simulink model "q_heli3d_w_ads"  (Simulink 7.7)
settings: Solver=ode1  StartTime=0.0  StopTime=inf  FixedStep=0.002  RelTol=1e-3
values from neighbouring files (symbols this model uses):
  CAL_TIME = 1.0    (= 1)    [setup_ads_configuration.m]
  CAL_VEL = 0.02    [setup_ads_configuration.m]
  CMD_ELEV_POS_LIMIT_LOWER = elev_0*180/pi    (= -27.5)    [setup_lab_heli_3d.m]    (also in setup_lab_heli_3d_simple.m; setup_lab_heli_3d_various_controler.m; setup_lab_heli_3d_various_controler_with_Kalman_Filter.m)
  CMD_ELEV_POS_LIMIT_UPPER = -CMD_ELEV_POS_LIMIT_LOWER    (= 27.5)    [setup_lab_heli_3d.m]    (also in setup_lab_heli_3d_simple.m; setup_lab_heli_3d_various_controler.m; setup_lab_heli_3d_various_controler_with_Kalman_Filter.m)
  CMD_RATE_LIMIT = 45.0 * pi / 180    (= 0.785398163397)    [setup_lab_heli_3d.m]    (also in setup_lab_heli_3d_simple.m; setup_lab_heli_3d_various_controler.m; setup_lab_heli_3d_various_controler_with_Kalman_Filter.m)
  elev_0 = -27.5*pi/180    (= -0.479965544298)    [setup_lab_heli_3d.m]    (also in setup_lab_heli_3d_simple.m; setup_lab_heli_3d_various_controler.m; setup_lab_heli_3d_various_controler_with_Kalman_Filter.m)
  g = 9.81    [linnlsys.m]
  K = lqr(A,B,Q_x,Q_u)    [lab_init.m]    (also in setup_lab_heli_3d.m = zeros(2,6); setup_lab_heli_3d_various_controler.m = lqr( Ai, Bi, Q, R ); setup_lab_heli_3d_various_controler_with_Kalman_Filter.m = lqr( Ai, Bi, Q, R ))
  K_AMP = 3    [setup_lab_heli_3d.m]    (also in setup_lab_heli_3d_simple.m; setup_lab_heli_3d_various_controler.m; setup_lab_heli_3d_various_controler_with_Kalman_Filter.m)
  K_AMP_X = 3    [setup_lab_heli_3d.m]    (also in setup_lab_heli_3d_simple.m; setup_lab_heli_3d_various_controler.m; setup_lab_heli_3d_various_controler_with_Kalman_Filter.m)
  K_JOYSTICK_X = 40.0    (= 40)    [setup_lab_heli_3d.m]    (also in setup_lab_heli_3d_simple.m; setup_lab_heli_3d_various_controler.m; setup_lab_heli_3d_various_controler_with_Kalman_Filter.m)
  K_JOYSTICK_Y = 45.0    (= 45)    [setup_lab_heli_3d.m]    (also in setup_lab_heli_3d_simple.m; setup_lab_heli_3d_various_controler.m; setup_lab_heli_3d_various_controler_with_Kalman_Filter.m)
  kp = 225    [setup_ads_configuration.m]
  La = 26.0 * 0.0254    (= 0.6604)    [linnlsys.m]
  POS_HOME = 11 * 0.0254 / 2    (= 0.1397)    [setup_ads_configuration.m]
  SAT_INT_ERR_ELEV = 7.5    [setup_lab_heli_3d.m]    (also in setup_lab_heli_3d_simple.m; setup_lab_heli_3d_various_controler.m; setup_lab_heli_3d_various_controler_with_Kalman_Filter.m)
  SAT_INT_ERR_TRAVEL = 7.5    [setup_lab_heli_3d.m]    (also in setup_lab_heli_3d_simple.m; setup_lab_heli_3d_various_controler.m; setup_lab_heli_3d_various_controler_with_Kalman_Filter.m)
  V_MAX = 0.08    [setup_ads_configuration.m]
  VMAX_AMP = 24    [setup_lab_heli_3d.m]    (also in setup_lab_heli_3d_simple.m; setup_lab_heli_3d_various_controler.m; setup_lab_heli_3d_various_controler_with_Kalman_Filter.m)
  VMAX_AMP_X = 15    [setup_lab_heli_3d.m]    (also in setup_lab_heli_3d_simple.m; setup_lab_heli_3d_various_controler.m; setup_lab_heli_3d_various_controler_with_Kalman_Filter.m)
  VMAX_DAC = 10    [setup_lab_heli_3d.m]    (also in setup_lab_heli_3d_simple.m; setup_lab_heli_3d_various_controler.m; setup_lab_heli_3d_various_controler_with_Kalman_Filter.m)
  wcf = 2 * pi * 2.5    (= 15.7079632679)    [setup_ads_configuration.m]    (also in setup_lab_heli_3d.m = 125.663706144; setup_lab_heli_3d_simple.m = 125.663706144; setup_lab_heli_3d_various_controler.m = 125.663706144; setup_lab_heli_3d_various_controler_with_Kalman_Filter.m = 125.663706144)
  X_MAX = 11 * 0.024    (= 0.264)    [setup_ads_configuration.m]
  zetaf = 0.9    [setup_lab_heli_3d.m]    (also in setup_lab_heli_3d_simple.m; setup_lab_heli_3d_various_controler.m; setup_lab_heli_3d_various_controler_with_Kalman_Filter.m)
undefined symbols (not defined in the file or in its folder): CMD_TRAVEL_POS_LIMIT_LOWER, CMD_TRAVEL_POS_LIMIT_UPPER, HIL, K_EC_E, K_EC_P, K_EC_T, K_EC_X, Kf, Lw, m_b, m_f, m_w, qc_get_step_size, wcf_x
libraries: quarc_library x6, simulink_extras x5, simulink x4
settings Model: Creator=MLevis  LastModifiedBy=MLevis  SimulationMode=external  ExtModeTrigDuration=5000
settings SolverCC: PositivePriorityOrder=on
settings OptimizationCC: InitFltsAndDblsToZero=on
settings DebuggingCC: SaveWithParameterizedLinksMsg=none  StrictBusMsg=Warning
settings RTWCC: SystemTargetFile=quarc_windows.tlc  TemplateMakefile=quarc_default_tmf  Description=QUARC Win32 Target  ProcessScript=quarc_windows_make_rtw_hook
settings STFCustomTargetCC: TargetFcnLib=ansi_tfl_tmw.mat  TargetPreCompLibLocation=C:\PROGRA~3\QUARC\lib\2011a\windows\release  FunctionExecutionProfile=off  GeneratePreprocessorConditionals=Disable all  SystemTargetFile=quarc_windows.tlc
settings GRTTargetCC: TargetFcnLib=ansi_tfl_tmw.mat  TargetPreCompLibLocation=C:\PROGRA~3\QUARC\lib\2011a\windows\release  ParMdlRefBuildCompliant=off  CompOptLevelCompliant=off  MatFileLogging=off  ExtMode=on  ExtModeMexFile=quarc_comm

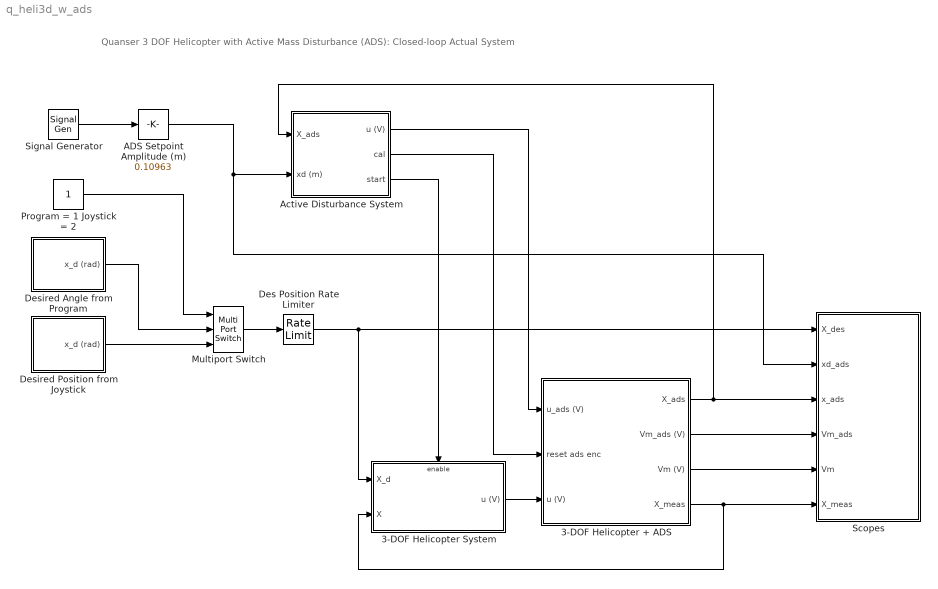
== system q_heli3d_w_ads ==
  note: Quanser 3 DOF Helicopter with Active Mass Disturbance (ADS):
      | Closed-loop Actual System
  3-DOF Helicopter + ADS : Subsystem
  3-DOF Helicopter System : Subsystem
  ADS Setpoint Amplitude (m) : simulink/Math Operations/Slider Gain  SystemSampleTime=-1  low=0  gain=0.10963  high=0.13
  Active Disturbance System : Subsystem
  Des Position Rate Limiter : RateLimiter  RisingSlewLimit=CMD_RATE_LIMIT  FallingSlewLimit=-CMD_RATE_LIMIT  SampleTimeMode=inherited
  Desired Angle from Program : Subsystem
  Desired Position from Joystick : Subsystem
  Multiport Switch : MultiPortSwitch  Inputs=2  zeroidx=off
  Program = 1 Joystick = 2 : Constant
  Scopes : Subsystem
  Signal Generator : SignalGenerator  WaveForm=square  Frequency=0.05
  wires:
  Signal Generator/1 -> ADS Setpoint Amplitude (m)/1
  ADS Setpoint Amplitude (m)/1 -> Scopes/2(xd_ads), Active Disturbance System/2(xd (m))
  Program = 1 Joystick = 2/1 -> Multiport Switch/1
  Desired Angle from Program/1(x_d (rad)) -> Multiport Switch/2
  Multiport Switch/1 -> Des Position Rate Limiter/1
  Desired Position from Joystick/1(x_d (rad)) -> Multiport Switch/3
  Des Position Rate Limiter/1 -> Scopes/1(X_des), 3-DOF Helicopter System/1(X_d)
  3-DOF Helicopter System/1(u (V)) -> 3-DOF Helicopter + ADS/3(u (V))
  Active Disturbance System/1(u (V)) -> 3-DOF Helicopter + ADS/1(u_ads (V))
  Active Disturbance System/2(cal) -> 3-DOF Helicopter + ADS/2(reset ads enc)
  3-DOF Helicopter + ADS/3(Vm (V)) -> Scopes/5(Vm)
  3-DOF Helicopter + ADS/4(X_meas) -> 3-DOF Helicopter System/2(X), Scopes/6(X_meas)
  3-DOF Helicopter + ADS/1(X_ads) -> Scopes/3(x_ads), Active Disturbance System/1(X_ads)
  Active Disturbance System/3(start) -> 3-DOF Helicopter System/Enable
  3-DOF Helicopter + ADS/2(Vm_ads (V)) -> Scopes/4(Vm_ads)

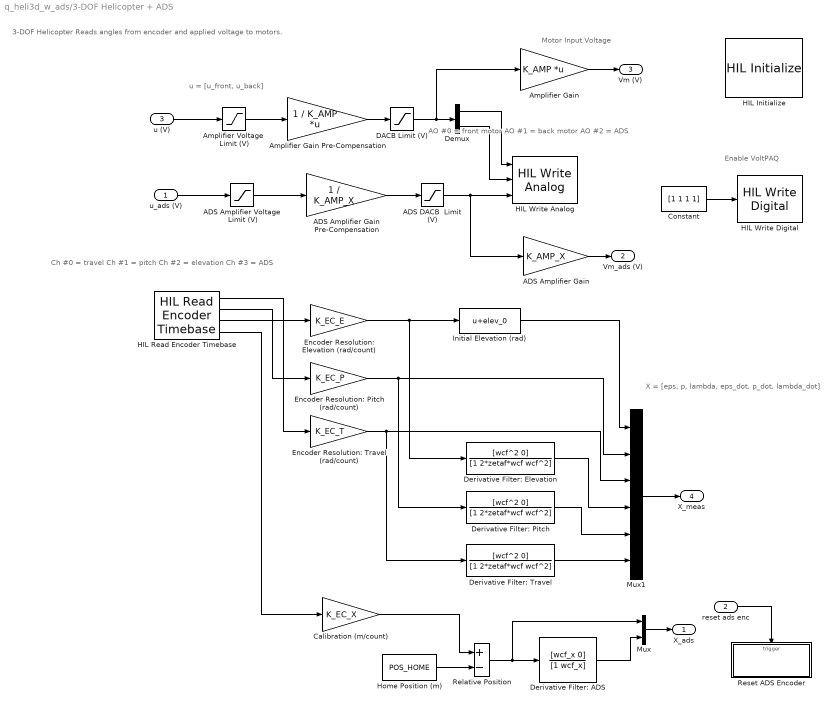
== system q_heli3d_w_ads/3-DOF Helicopter + ADS ==
  note: Enable VoltPAQ
  note: X = [eps, p, lambda, eps_dot, p_dot, lambda_dot]
  note: Ch #0 = travel
      | Ch #1 = pitch
      | Ch #2 = elevation
      | Ch #3 = ADS
  note: 3-DOF Helicopter
      | Reads angles from encoder and applied voltage to motors.
  note: Motor Input Voltage
  note: u = [u_front, u_back]
  note: AO #0 = front motor
      | AO #1 = back motor
      | AO #2 = ADS
  u_ads (V) : Inport
  reset ads enc : Inport  Port=2
  u (V) : Inport  Port=3
  ADS Amplifier Gain : Gain  Gain=K_AMP_X  SaturateOnIntegerOverflow=on  OutDataTypeStr=Inherit: Same as input  ParamDataTypeStr=Inherit: Same as input
  ADS Amplifier Gain Pre-Compensation : Gain  Gain=1 / K_AMP_X  SaturateOnIntegerOverflow=on  OutDataTypeStr=Inherit: Same as input  ParamDataTypeStr=Inherit: Same as input
  ADS Amplifier Voltage  Limit (V) : Saturate  UpperLimit=VMAX_AMP_X  LowerLimit=-VMAX_AMP_X
  ADS DACB  Limit (V) : Saturate  UpperLimit=VMAX_DAC  LowerLimit=-VMAX_DAC
  Amplifier Gain : Gain  Gain=K_AMP  Multiplication=Matrix(K*u)  SaturateOnIntegerOverflow=on  OutDataTypeStr=Inherit: Same as input  ParamDataTypeStr=Inherit: Same as input
  Amplifier Gain Pre-Compensation : Gain  Gain=1 / K_AMP  Multiplication=Matrix(K*u)  SaturateOnIntegerOverflow=on  OutDataTypeStr=Inherit: Same as input  ParamDataTypeStr=Inherit: Same as input
  Amplifier Voltage  Limit (V) : Saturate  UpperLimit=VMAX_AMP  LowerLimit=-VMAX_AMP
  Calibration (m/count) : Gain  Gain=K_EC_X  SaturateOnIntegerOverflow=on  OutDataTypeStr=Inherit: Same as input  ParamDataTypeStr=Inherit: Same as input
  Constant : Constant  Value=[1 1 1 1]
  DACB Limit (V) : Saturate  UpperLimit=VMAX_DAC  LowerLimit=-VMAX_DAC
  Demux : Demux  Outputs=2
  Derivative Filter: ADS : TransferFcn  Numerator=[wcf_x 0]  Denominator=[1 wcf_x]
  Derivative Filter: Elevation : TransferFcn  Numerator=[wcf^2 0]  Denominator=[1 2*zetaf*wcf wcf^2]
  Derivative Filter: Pitch : TransferFcn  Numerator=[wcf^2 0]  Denominator=[1 2*zetaf*wcf wcf^2]
  Derivative Filter: Travel : TransferFcn  Numerator=[wcf^2 0]  Denominator=[1 2*zetaf*wcf wcf^2]
  Encoder Resolution: Elevation (rad/count) : Gain  Gain=K_EC_E
  Encoder Resolution: Pitch (rad/count) : Gain  Gain=K_EC_P
  Encoder Resolution: Travel (rad/count) : Gain  Gain=K_EC_T
  HIL Initialize : quarc_library/Data Acquisition/Generic/Configuration/HIL Initialize  object_name=HIL-1  board_type=q8_usb  board_number=0  board_options=update_rate=normal  exclusive=off  active=on  hardware_clocks=[0:2]  clock_modes=[]  initial_clock_frequencies=[]  set_clock_params_at_start=off  set_clock_params_at_switch_in=off  set_clock_frequencies_at_start=off  set_clock_frequencies_at_switch_in=off  analog_input_channels=[0:7]  analog_input_maximums=10  analog_input_minimums=-10  set_analog_input_params_at_start=on  set_analog_input_params_at_switch_in=off  analog_output_channels=[0:7]  analog_output_maximums=10  analog_output_minimums=-10  initial_analog_outputs=[0]  final_analog_outputs=[0]  watchdog_analog_outputs=0  set_analog_output_params_at_start=on  set_analog_output_params_at_switch_in=off  set_analog_outputs_at_start=on  set_analog_outputs_at_switch_in=off  set_analog_outputs_at_terminate=on  set_analog_outputs_at_switch_out=off  set_analog_outputs_on_watchdog=off  digital_input_channels=[]  digital_output_channels=[0:2]  digital_output_configuration=[]  initial_digital_outputs=[0 0 0]  final_digital_outputs=[0 0 0]  watchdog_digital_outputs=[1]  set_digital_output_params_at_start=off  set_digital_output_params_at_switch_in=off  set_digital_outputs_at_start=on  set_digital_outputs_at_switch_in=off  set_digital_outputs_at_terminate=on  set_digital_outputs_at_switch_out=off  set_digital_outputs_on_watchdog=off  encoder_channels=[0:7]  quadrature=[4]  encoder_filter_frequency=[]  initial_encoder_counts=[0]  set_encoder_params_at_start=on  set_encoder_params_at_switch_in=off  set_encoder_counts_at_start=on  set_encoder_counts_at_switch_in=off  pwm_channels=[0:7]  pwm_modes=0  pwm_frequency=99.532799999999995e6/4095  pwm_configuration=[0]  pwm_alignment=[0]  pwm_polarity=[1]  pwm_leading_deadband=[0]  pwm_trailing_deadband=[0]  initial_pwm_outputs=[0]  final_pwm_outputs=[0]  watchdog_pwm_outputs=[0]  set_pwm_params_at_start=on  set_pwm_params_at_switch_in=off  set_pwm_outputs_at_start=on  set_pwm_outputs_at_switch_in=off  set_pwm_outputs_at_terminate=on  set_pwm_outputs_at_switch_out=off  set_pwm_outputs_on_watchdog=off  other_output_channels=[]  initial_other_outputs=[]  final_other_outputs=[]  watchdog_other_outputs=[]  set_other_outputs_at_start=off  set_other_outputs_at_switch_in=off  set_other_outputs_at_terminate=off  set_other_outputs_at_switch_out=off  set_other_outputs_on_watchdog=off
  HIL Read Encoder Timebase : quarc_library/Data Acquisition/Generic/Timebases/HIL Read Encoder Timebase  object_name=HIL-1  clock=0  channels=[0:3]  samples_in_buffer=max(ceil(1/qc_get_step_size), 1)  active=on  vector_output=off  data_type_mode=Inherit via back propagation  data_type=double
  HIL Write Analog : quarc_library/Data Acquisition/Generic/Immediate I//O/HIL Write Analog  object_name=HIL-1  channels=[0:2]  sample_time=-1  active=off  vector_input=off
  HIL Write Digital : quarc_library/Data Acquisition/Generic/Immediate I//O/HIL Write Digital  object_name=HIL-1  channels=[0:3]  sample_time=-1  active=off  vector_input=on
  Home Position (m) : Constant  Value=POS_HOME
  Initial Elevation (rad) : Bias  Bias=elev_0
  Mux : Mux  Inputs=2
  Mux1 : Mux  Inputs=6
  Relative Position : Sum  Inputs=+-  SaturateOnIntegerOverflow=on  InputSameDT=on  OutDataTypeStr=Inherit: Same as first input
  Reset ADS Encoder : Subsystem  TreatAsAtomicUnit=on
  X_ads : Outport
  Vm_ads (V) : Outport  Port=2
  Vm (V) : Outport  Port=3
  X_meas : Outport  Port=4
  wires:
  Constant/1 -> HIL Write Digital/1
  Mux/1 -> X_ads/1
  Initial Elevation (rad)/1 -> Mux1/1
  Derivative Filter: Travel/1 -> Mux1/6
  Derivative Filter: Pitch/1 -> Mux1/5
  Derivative Filter: Elevation/1 -> Mux1/4
  Encoder Resolution: Travel (rad/count)/1 -> Derivative Filter: Travel/1, Mux1/3
  Encoder Resolution: Pitch (rad/count)/1 -> Derivative Filter: Pitch/1, Mux1/2
  Encoder Resolution: Elevation (rad/count)/1 -> Initial Elevation (rad)/1, Derivative Filter: Elevation/1
  HIL Read Encoder Timebase/2 -> Encoder Resolution: Pitch (rad/count)/1
  HIL Read Encoder Timebase/1 -> Encoder Resolution: Travel (rad/count)/1
  HIL Read Encoder Timebase/3 -> Encoder Resolution: Elevation (rad/count)/1
  DACB Limit (V)/1 -> Amplifier Gain/1, Demux/1
  u (V)/1 -> Amplifier Voltage  Limit (V)/1
  Amplifier Gain/1 -> Vm (V)/1
  Amplifier Voltage  Limit (V)/1 -> Amplifier Gain Pre-Compensation/1
  Amplifier Gain Pre-Compensation/1 -> DACB Limit (V)/1
  Mux1/1 -> X_meas/1
  HIL Read Encoder Timebase/4 -> Calibration (m/count)/1
  Calibration (m/count)/1 -> Relative Position/1
  Home Position (m)/1 -> Relative Position/2
  Derivative Filter: ADS/1 -> Mux/2
  Relative Position/1 -> Mux/1, Derivative Filter: ADS/1
  Demux/1 -> HIL Write Analog/1
  Demux/2 -> HIL Write Analog/2
  ADS Amplifier Gain Pre-Compensation/1 -> ADS DACB  Limit (V)/1
  ADS Amplifier Voltage  Limit (V)/1 -> ADS Amplifier Gain Pre-Compensation/1
  u_ads (V)/1 -> ADS Amplifier Voltage  Limit (V)/1
  ADS DACB  Limit (V)/1 -> HIL Write Analog/3, ADS Amplifier Gain/1
  ADS Amplifier Gain/1 -> Vm_ads (V)/1
  reset ads enc/1 -> Reset ADS Encoder/Trigger

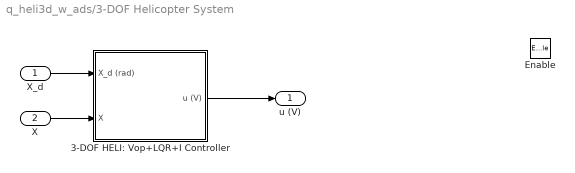
== system q_heli3d_w_ads/3-DOF Helicopter System ==
  X_d : Inport
  X : Inport  Port=2
  Enable : EnablePort
  3-DOF HELI: Vop+LQR+I Controller : Subsystem
  u (V) : Outport  OutputWhenDisabled=reset  InitialOutput=[0,0]
  wires:
  X/1 -> 3-DOF HELI: Vop+LQR+I Controller/2(X)
  3-DOF HELI: Vop+LQR+I Controller/1(u (V)) -> u (V)/1
  X_d/1 -> 3-DOF HELI: Vop+LQR+I Controller/1(X_d (rad))

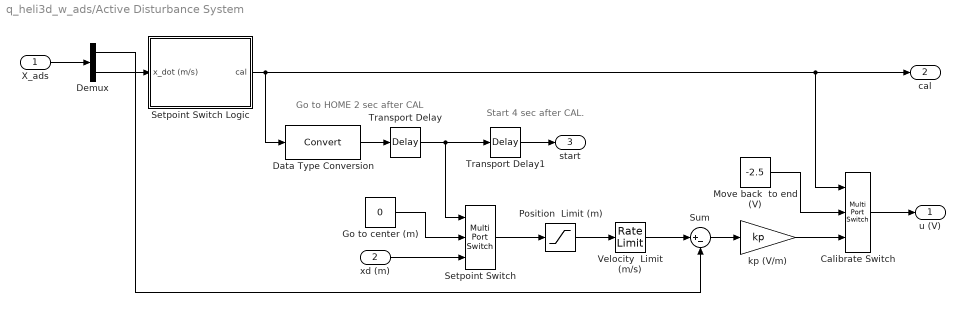
== system q_heli3d_w_ads/Active Disturbance System ==
  note: Start 4 sec after CAL.
  note: Go to HOME 2 sec
      | after CAL
  X_ads : Inport
  xd (m) : Inport  Port=2
  Calibrate Switch : MultiPortSwitch  DataPortOrder=Zero-based contiguous  Inputs=2  zeroidx=on  SaturateOnIntegerOverflow=on  InputSameDT=on
  Data Type Conversion : DataTypeConversion
  Demux : Demux  Outputs=2
  Go to center (m) : Constant  Value=0
  Move back  to end (V) : Constant  Value=-2.5
  Position  Limit (m) : Saturate  UpperLimit=X_MAX  LowerLimit=-X_MAX
  Setpoint Switch : MultiPortSwitch  DataPortOrder=Zero-based contiguous  Inputs=2  zeroidx=on  SampleTime=qc_get_step_size  SaturateOnIntegerOverflow=on  InputSameDT=on
  Setpoint Switch Logic : Subsystem
  Sum : Sum  Inputs=|+-
  Transport Delay : TransportDelay  DelayTime=2
  Transport Delay1 : TransportDelay  DelayTime=2
  Velocity  Limit (m/s) : RateLimiter  RisingSlewLimit=V_MAX  FallingSlewLimit=-V_MAX
  kp (V/m) : Gain  Gain=kp  SaturateOnIntegerOverflow=on  OutDataTypeStr=Inherit: Same as input  ParamDataTypeStr=Inherit: Same as input
  u (V) : Outport
  cal : Outport  Port=2
  start : Outport  Port=3
  wires:
  Demux/2 -> Setpoint Switch Logic/1(x_dot (m/s))
  Demux/1 -> Sum/2
  X_ads/1 -> Demux/1
  kp (V/m)/1 -> Calibrate Switch/3
  Velocity  Limit (m/s)/1 -> Sum/1
  Calibrate Switch/1 -> u (V)/1
  Data Type Conversion/1 -> Transport Delay/1
  Position  Limit (m)/1 -> Velocity  Limit (m/s)/1
  Setpoint Switch Logic/1(cal) -> cal/1, Calibrate Switch/1, Data Type Conversion/1
  Go to center (m)/1 -> Setpoint Switch/2
  Sum/1 -> kp (V/m)/1
  Move back  to end (V)/1 -> Calibrate Switch/2
  Transport Delay/1 -> Transport Delay1/1, Setpoint Switch/1
  xd (m)/1 -> Setpoint Switch/3
  Transport Delay1/1 -> start/1
  Setpoint Switch/1 -> Position  Limit (m)/1

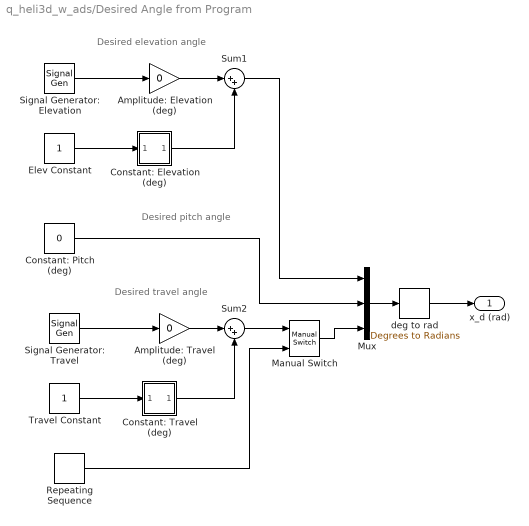
== system q_heli3d_w_ads/Desired Angle from Program ==
  note: Desired pitch angle
  note: Desired elevation angle
  note: Desired travel angle
  Amplitude: Elevation (deg) : Gain  Gain=0
  Amplitude: Travel (deg) : Gain  Gain=0
  Constant: Elevation (deg) : Subsystem  LoadFcn=slideg Load  StartFcn=slideg StartFcn  StopFcn=slideg StopFcn  mask(Slider Gain){low=-27.5, gain=-27.5, high=30}
      settings: CopyFcn=slideg Copy  DeleteFcn=slideg DeleteBlock  NameChangeFcn=slideg NameChange  OpenFcn=slideg Open  CloseFcn=slideg Close  ParentCloseFcn=slideg ParentClose
      mask Display: disp(gain)
  Constant: Pitch (deg) : Constant  Value=0
  Constant: Travel (deg) : Subsystem  LoadFcn=slideg Load  StartFcn=slideg StartFcn  StopFcn=slideg StopFcn  mask(Slider Gain){low=-90, gain=0, high=90}
      settings: CopyFcn=slideg Copy  DeleteFcn=slideg DeleteBlock  NameChangeFcn=slideg NameChange  OpenFcn=slideg Open  CloseFcn=slideg Close  ParentCloseFcn=slideg ParentClose
      mask Display: disp(gain)
  Elev Constant : Constant
  Manual Switch : simulink/Signal Routing/Manual Switch  SystemSampleTime=-1  sw=1  action=0  varsize=off
  Mux : Mux  Inputs=3
  Repeating Sequence : simulink/Sources/Repeating Sequence  SystemSampleTime=-1  rep_seq_t="[0  15 16  30  45  46 60 ]"  rep_seq_y="[0 0 30 30  30 0 0 ]"
  Signal Generator: Elevation : SignalGenerator  WaveForm=square  Frequency=0.04
  Signal Generator: Travel : SignalGenerator  WaveForm=square  Frequency=0.03
  Sum1 : Sum  Inputs=|++
  Sum2 : Sum  Inputs=|++
  Travel Constant : Constant
  deg to rad : simulink_extras/Transformations/Degrees to Radians  SystemSampleTime=-1
  x_d (rad) : Outport
  wires:
  Repeating Sequence/1 -> Manual Switch/2
  Manual Switch/1 -> Mux/3
  Sum2/1 -> Manual Switch/1
  Constant: Travel (deg)/1(Out1) -> Sum2/2
  Constant: Elevation (deg)/1(Out1) -> Sum1/2
  Elev Constant/1 -> Constant: Elevation (deg)/1(In1)
  Constant: Pitch (deg)/1 -> Mux/2
  Mux/1 -> deg to rad/1
  Amplitude: Elevation (deg)/1 -> Sum1/1
  Signal Generator: Elevation/1 -> Amplitude: Elevation (deg)/1
  Sum1/1 -> Mux/1
  Travel Constant/1 -> Constant: Travel (deg)/1(In1)
  Amplitude: Travel (deg)/1 -> Sum2/1
  Signal Generator: Travel/1 -> Amplitude: Travel (deg)/1
  deg to rad/1 -> x_d (rad)/1

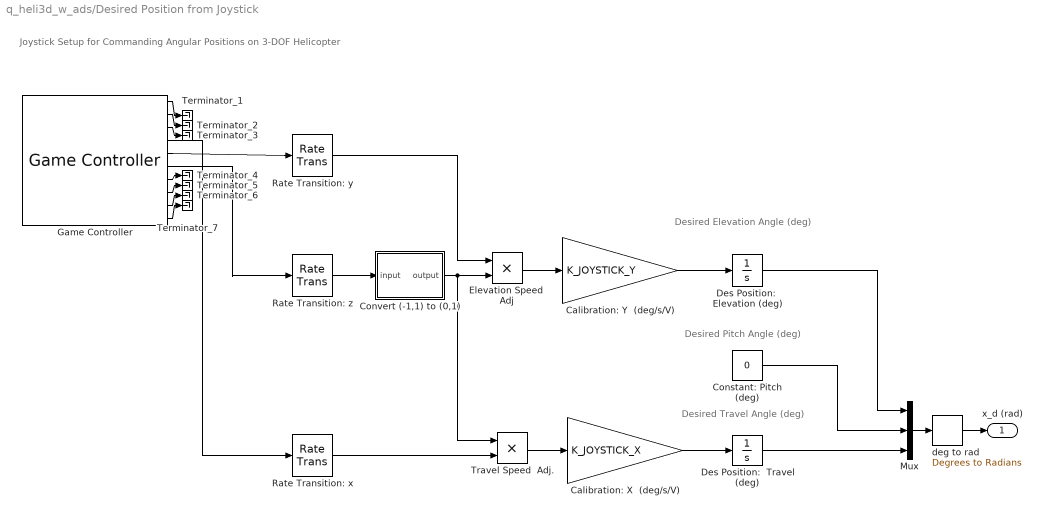
== system q_heli3d_w_ads/Desired Position from Joystick ==
  note: Joystick Setup for Commanding Angular Positions on 3-DOF Helicopter
  note: Desired Travel Angle (deg)
  note: Desired Elevation Angle (deg)
  note: Desired Pitch Angle (deg)
  Calibration: X  (deg/s/V) : Gain  Gain=K_JOYSTICK_X
  Calibration: Y  (deg/s/V) : Gain  Gain=K_JOYSTICK_Y
  Constant: Pitch (deg) : Constant  Value=0
  Convert (-1,1) to (0,1) : Subsystem
  Des Position:  Elevation (deg) : Integrator  InitialCondition=elev_0*180/pi  LimitOutput=on  UpperSaturationLimit=CMD_ELEV_POS_LIMIT_UPPER  LowerSaturationLimit=CMD_ELEV_POS_LIMIT_LOWER
  Des Position:  Travel (deg) : Integrator  UpperSaturationLimit=CMD_TRAVEL_POS_LIMIT_UPPER  LowerSaturationLimit=CMD_TRAVEL_POS_LIMIT_LOWER
  Elevation Speed  Adj : Product  RndMeth=Zero
  Game Controller : quarc_library/Devices/Peripherals/Target/Game Controller  controller=1  buffer_size=12  deadzone=[]  saturation=[]  sample_time=max(qc_get_step_size, 0.01)  auto_center=off  enabled=on
  Mux : Mux  Inputs=3
  Rate Transition: x : RateTransition
  Rate Transition: y : RateTransition
  Rate Transition: z : RateTransition
  Terminator_{1..7} (7 alike) : Terminator
  Travel Speed  Adj. : Product  RndMeth=Zero
  deg to rad : simulink_extras/Transformations/Degrees to Radians  SystemSampleTime=-1
  x_d (rad) : Outport
  wires:
  Game Controller/10 -> Terminator_7/1
  Game Controller/9 -> Terminator_6/1
  Game Controller/8 -> Terminator_5/1
  Game Controller/7 -> Terminator_4/1
  Game Controller/3 -> Terminator_3/1
  Game Controller/2 -> Terminator_2/1
  Game Controller/1 -> Terminator_1/1
  Game Controller/4 -> Rate Transition: x/1
  Game Controller/6 -> Rate Transition: z/1
  Game Controller/5 -> Rate Transition: y/1
  Rate Transition: x/1 -> Travel Speed  Adj./2
  Rate Transition: y/1 -> Elevation Speed  Adj/1
  Rate Transition: z/1 -> Convert (-1,1) to (0,1)/1(input)
  Convert (-1,1) to (0,1)/1(output) -> Elevation Speed  Adj/2, Travel Speed  Adj./1
  Calibration: Y  (deg/s/V)/1 -> Des Position:  Elevation (deg)/1
  Elevation Speed  Adj/1 -> Calibration: Y  (deg/s/V)/1
  Travel Speed  Adj./1 -> Calibration: X  (deg/s/V)/1
  Calibration: X  (deg/s/V)/1 -> Des Position:  Travel (deg)/1
  deg to rad/1 -> x_d (rad)/1
  Mux/1 -> deg to rad/1
  Des Position:  Travel (deg)/1 -> Mux/3
  Constant: Pitch (deg)/1 -> Mux/2
  Des Position:  Elevation (deg)/1 -> Mux/1

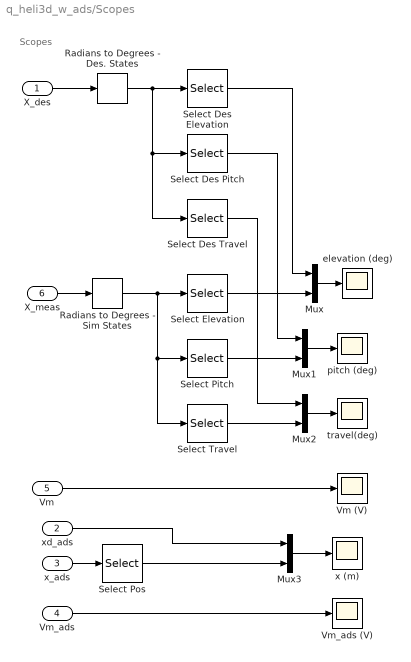
== system q_heli3d_w_ads/Scopes ==
  note: Scopes
  X_des : Inport
  xd_ads : Inport  Port=2
  x_ads : Inport  Port=3
  Vm_ads : Inport  Port=4
  Vm : Inport  Port=5
  X_meas : Inport  Port=6
  Mux{,1..3} (4 alike) : Mux  Inputs=2
  Radians to Degrees - Des. States : simulink_extras/Transformations/Radians to Degrees  SystemSampleTime=-1
  Radians to Degrees - Sim States : simulink_extras/Transformations/Radians to Degrees  SystemSampleTime=-1
  Select Des Elevation : Selector  InputPortWidth=3  IndexOptions=Index vector (dialog)  Indices=1  OutputSizes=1
  Select Des Pitch : Selector  InputPortWidth=3  IndexOptions=Index vector (dialog)  Indices=2  OutputSizes=1
  Select Des Travel : Selector  InputPortWidth=3  IndexOptions=Index vector (dialog)  Indices=3  OutputSizes=1
  Select Elevation : Selector  InputPortWidth=6  IndexOptions=Index vector (dialog)  Indices=1  OutputSizes=1
  Select Pitch : Selector  InputPortWidth=6  IndexOptions=Index vector (dialog)  Indices=2  OutputSizes=1
  Select Pos : Selector  InputPortWidth=2  IndexOptions=Index vector (dialog)  Indices=1  OutputSizes=1
  Select Travel : Selector  InputPortWidth=6  IndexOptions=Index vector (dialog)  Indices=3  OutputSizes=1
  Vm (V) : Scope
      settings: TickLabels=on  TimeRange=20  YMin=0  YMax=18  SaveName=ScopeData4  DataFormat=Array
  Vm_ads (V) : Scope
      settings: TickLabels=on  TimeRange=20  YMin=0  YMax=18  SaveName=ScopeData3  DataFormat=Array
  elevation (deg) : Scope
      settings: TickLabels=on  TimeRange=20  YMin=-15  YMax=15  DataFormat=Array
  pitch (deg) : Scope
      settings: TickLabels=on  TimeRange=20  YMin=-80  YMax=80  DataFormat=Array
  travel(deg) : Scope
      settings: TickLabels=on  TimeRange=20  YMin=-80  YMax=80  SaveName=ScopeData2  DataFormat=Array
  x (m) : Scope
      settings: YMin=-0.15  YMax=0.15  SaveName=ScopeData5
  wires:
  Select Pos/1 -> Mux3/2
  Vm_ads/1 -> Vm_ads (V)/1
  Mux3/1 -> x (m)/1
  x_ads/1 -> Select Pos/1
  xd_ads/1 -> Mux3/1
  Select Des Travel/1 -> Mux2/1
  Select Des Pitch/1 -> Mux1/1
  Select Des Elevation/1 -> Mux/1
  Radians to Degrees - Des. States/1 -> Select Des Travel/1, Select Des Pitch/1, Select Des Elevation/1
  Select Travel/1 -> Mux2/2
  Select Pitch/1 -> Mux1/2
  Select Elevation/1 -> Mux/2
  Mux2/1 -> travel(deg)/1
  Radians to Degrees - Sim States/1 -> Select Travel/1, Select Pitch/1, Select Elevation/1
  Vm/1 -> Vm (V)/1
  Mux1/1 -> pitch (deg)/1
  Mux/1 -> elevation (deg)/1
  X_meas/1 -> Radians to Degrees - Sim States/1
  X_des/1 -> Radians to Degrees - Des. States/1

== system q_heli3d_w_ads/3-DOF Helicopter + ADS/Reset ADS Encoder ==
  Trigger : TriggerPort
  HIL Set Encoder Counts : quarc_library/Data Acquisition/Generic/Configuration/HIL Set Encoder Counts  object_name=HIL-1  channels=3  source=internal  counts=0  sample_time=-1  active=on  vector_input=off
      settings: AttributesFormatString=(%<object_name>)

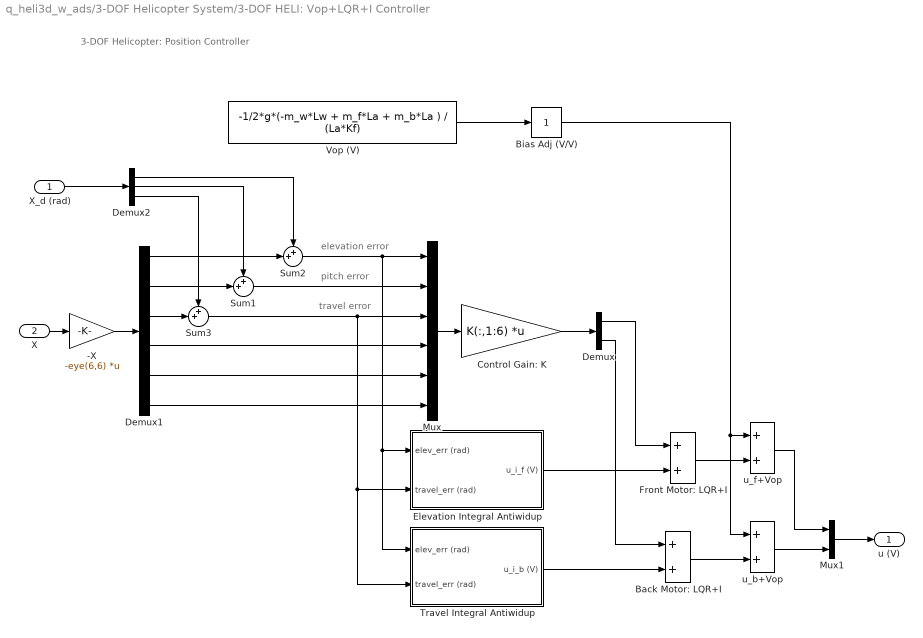
== system q_heli3d_w_ads/3-DOF Helicopter System/3-DOF HELI: Vop+LQR+I Controller ==
  note: travel error
  note: 3-DOF Helicopter: Position Controller
  note: pitch error
  note: elevation error
  X_d (rad) : Inport
  X : Inport  Port=2
  -X : Gain  Gain=-eye(6,6)  Multiplication=Matrix(K*u)
  Back Motor: LQR+I : Sum
  Bias Adj (V/V) : simulink/Math Operations/Slider Gain  SystemSampleTime=-1  low=0  gain=1  high=1
  Control Gain: K : Gain  Gain=K(:,1:6)  Multiplication=Matrix(K*u)
  Demux : Demux  Outputs=2
  Demux1 : Demux  Outputs=6
  Demux2 : Demux  Outputs=3
  Elevation Integral Antiwidup : Subsystem
  Front Motor: LQR+I : Sum
  Mux : Mux  Inputs=6
  Mux1 : Mux  Inputs=2
  Sum1 : Sum  Inputs=++|
  Sum2 : Sum  Inputs=++|
  Sum3 : Sum  Inputs=++|
  Travel Integral Antiwidup : Subsystem
  Vop (V) : Constant  Value=-1/2*g*(-m_w*Lw + m_f*La + m_b*La ) / (La*Kf)
  u_b+Vop : Sum
  u_f+Vop : Sum
  u (V) : Outport
  wires:
  Mux1/1 -> u (V)/1
  Control Gain: K/1 -> Demux/1
  Demux1/6 -> Mux/6
  Demux1/5 -> Mux/5
  Sum3/1 -> Travel Integral Antiwidup/2(travel_err (rad)), Elevation Integral Antiwidup/2(travel_err (rad)), Mux/3
  Demux1/3 -> Sum3/2
  Demux2/3 -> Sum3/1
  Demux1/4 -> Mux/4
  Mux/1 -> Control Gain: K/1
  -X/1 -> Demux1/1
  Sum1/1 -> Mux/2
  X/1 -> -X/1
  Demux1/1 -> Sum2/2
  Sum2/1 -> Travel Integral Antiwidup/1(elev_err (rad)), Elevation Integral Antiwidup/1(elev_err (rad)), Mux/1
  X_d (rad)/1 -> Demux2/1
  Demux2/1 -> Sum2/1
  Demux2/2 -> Sum1/1
  Demux1/2 -> Sum1/2
  Vop (V)/1 -> Bias Adj (V/V)/1
  Elevation Integral Antiwidup/1(u_i_f (V)) -> Front Motor: LQR+I/2
  Travel Integral Antiwidup/1(u_i_b (V)) -> Back Motor: LQR+I/2
  Demux/2 -> Back Motor: LQR+I/1
  Demux/1 -> Front Motor: LQR+I/1
  Front Motor: LQR+I/1 -> u_f+Vop/2
  Back Motor: LQR+I/1 -> u_b+Vop/2
  u_b+Vop/1 -> Mux1/2
  Bias Adj (V/V)/1 -> u_f+Vop/1, u_b+Vop/1
  u_f+Vop/1 -> Mux1/1

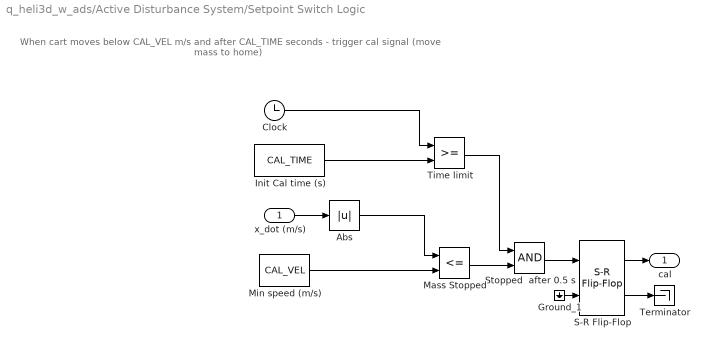
== system q_heli3d_w_ads/Active Disturbance System/Setpoint Switch Logic ==
  note: When cart moves below CAL_VEL m/s and after
      | CAL_TIME seconds - trigger cal signal (move mass to home)
  x_dot (m/s) : Inport
  Abs : Abs  SaturateOnIntegerOverflow=on
  Clock : Clock
      settings: Decimation=10
  Ground_1 : Ground
  Init Cal time (s) : Constant  Value=CAL_TIME
  Mass Stopped : RelationalOperator  Operator=<=  InputSameDT=on
  Min speed (m/s) : Constant  Value=CAL_VEL
  S-R Flip-Flop : simulink_extras/Flip Flops/S-R Flip-Flop  SystemSampleTime=-1  initial_condition=0
  Stopped  after 0.5 s : Logic
  Terminator : Terminator
  Time limit : RelationalOperator  InputSameDT=on
  cal : Outport
  wires:
  Ground_1/1 -> S-R Flip-Flop/2
  S-R Flip-Flop/2 -> Terminator/1
  x_dot (m/s)/1 -> Abs/1
  S-R Flip-Flop/1 -> cal/1
  Stopped  after 0.5 s/1 -> S-R Flip-Flop/1
  Clock/1 -> Time limit/1
  Time limit/1 -> Stopped  after 0.5 s/1
  Init Cal time (s)/1 -> Time limit/2
  Mass Stopped/1 -> Stopped  after 0.5 s/2
  Min speed (m/s)/1 -> Mass Stopped/2
  Abs/1 -> Mass Stopped/1

== system q_heli3d_w_ads/Desired Angle from Program/Constant: Elevation (deg) ==
  In1 : Inport
  Slider Gain : Gain  Gain=gain  SaturateOnIntegerOverflow=on  OutDataTypeStr=Inherit: Same as input  ParamDataTypeStr=Inherit: Same as input
  Out1 : Outport
  wires:
  Slider Gain/1 -> Out1/1
  In1/1 -> Slider Gain/1

== system q_heli3d_w_ads/Desired Angle from Program/Constant: Travel (deg) ==
  In1 : Inport
  Slider Gain : Gain  Gain=gain  SaturateOnIntegerOverflow=on  OutDataTypeStr=Inherit: Same as input  ParamDataTypeStr=Inherit: Same as input
  Out1 : Outport
  wires:
  Slider Gain/1 -> Out1/1
  In1/1 -> Slider Gain/1

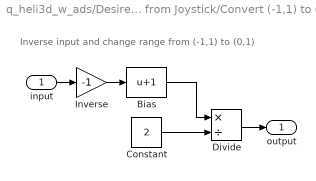
== system q_heli3d_w_ads/Desired Position from Joystick/Convert (-1,1) to (0,1) ==
  note: Inverse input and change range from (-1,1) to (0,1)
  input : Inport
  Bias : Bias  Bias=1
  Constant : Constant  Value=2
  Divide : Product  Inputs=*/
  Inverse : Gain  Gain=-1
  output : Outport
  wires:
  Inverse/1 -> Bias/1
  Divide/1 -> output/1
  input/1 -> Inverse/1
  Bias/1 -> Divide/1
  Constant/1 -> Divide/2

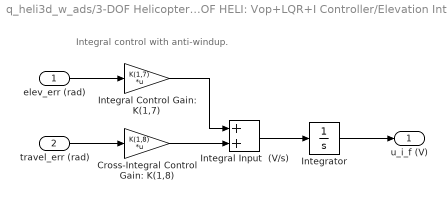
== system q_heli3d_w_ads/3-DOF Helicopter System/3-DOF HELI: Vop+LQR+I Controller/Elevation Integral Antiwidup ==
  note: Integral control with anti-windup.
  elev_err (rad) : Inport
  travel_err (rad) : Inport  Port=2
  Cross-Integral Control Gain: K(1,8) : Gain  Gain=K(1,8)  Multiplication=Matrix(K*u)
  Integral Control Gain: K(1,7) : Gain  Gain=K(1,7)  Multiplication=Matrix(K*u)
  Integral Input  (V/s) : Sum
  Integrator : Integrator  LimitOutput=on  UpperSaturationLimit=SAT_INT_ERR_ELEV  LowerSaturationLimit=-SAT_INT_ERR_ELEV
  u_i_f (V) : Outport
  wires:
  Integrator/1 -> u_i_f (V)/1
  Integral Input  (V/s)/1 -> Integrator/1
  elev_err (rad)/1 -> Integral Control Gain: K(1,7)/1
  travel_err (rad)/1 -> Cross-Integral Control Gain: K(1,8)/1
  Integral Control Gain: K(1,7)/1 -> Integral Input  (V/s)/1
  Cross-Integral Control Gain: K(1,8)/1 -> Integral Input  (V/s)/2

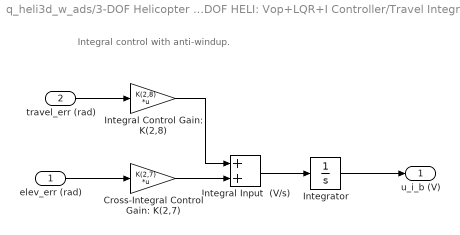
== system q_heli3d_w_ads/3-DOF Helicopter System/3-DOF HELI: Vop+LQR+I Controller/Travel Integral Antiwidup ==
  note: Integral control with anti-windup.
  elev_err (rad) : Inport
  travel_err (rad) : Inport  Port=2
  Cross-Integral Control Gain: K(2,7) : Gain  Gain=K(2,7)  Multiplication=Matrix(K*u)
  Integral Control Gain: K(2,8) : Gain  Gain=K(2,8)  Multiplication=Matrix(K*u)
  Integral Input  (V/s) : Sum
  Integrator : Integrator  LimitOutput=on  UpperSaturationLimit=SAT_INT_ERR_TRAVEL  LowerSaturationLimit=-SAT_INT_ERR_TRAVEL
  u_i_b (V) : Outport
  wires:
  Integrator/1 -> u_i_b (V)/1
  Integral Input  (V/s)/1 -> Integrator/1
  elev_err (rad)/1 -> Cross-Integral Control Gain: K(2,7)/1
  travel_err (rad)/1 -> Integral Control Gain: K(2,8)/1
  Integral Control Gain: K(2,8)/1 -> Integral Input  (V/s)/1
  Cross-Integral Control Gain: K(2,7)/1 -> Integral Input  (V/s)/2
